simulink model "SAR_ADC_Dom_14_04_2017"  (R2016a)
settings: Solver=ode45  StartTime=0.0  StopTime=inf  FixedStep=1/255/2  RelTol=1e-3
libraries: simulink_extras x10
settings Model: Creator=ronip  LastModifiedBy=Lara
settings SolverCC: AutoInsertRateTranBlk=on
settings DataIOCC: SaveFormat=Array  SignalLoggingSaveFormat=ModelDataLogs  SaveOutput=off  SignalLogging=off  DSMLogging=off  SaveTime=off
settings OptimizationCC: ExpressionDepthLimit=2147483647  StateBitsets=on  DataBitsets=on  OptimizeModelRefInitCode=on  LifeSpan=1
settings DebuggingCC: UnderspecifiedInitializationDetection=Classic  MergeDetectMultiDrivingBlocksExec=none  SolverPrmCheckMsg=warning  FcnCallInpInsideContextMsg=UseLocalSettings  BusObjectLabelMismatch=error  StateNameClashWarn=warning
settings HardwareCC: ProdBitPerPointer=32  ProdLargestAtomicFloat=None  ProdIntDivRoundTo=Undefined  ProdEndianess=Unspecified  ProdWordSize=32  ProdHWDeviceType=32-bit Generic
settings ModelReferenceCC: PropagateSignalLabelsOutOfModel=off
settings RTWCC: SystemTargetFile=ert.tlc  TemplateMakefile=ert_default_tmf  Description=Real-Time Workshop Embedded Coder  GenerateReport=on  IncludeHyperlinkInReport=on  LaunchReport=on  CreateSILPILBlock=SIL  GenerateTraceInfo=on  GenerateTraceReport=on  GenerateTraceReportSl=on  GenerateTraceReportSf=on  GenerateTraceReportEml=on
settings CodeAppCC: IgnoreCustomStorageClasses=off  CustomSymbolStrType=$N$R$M  InternalIdentifier=Classic
settings ERTTargetCC: GenerateSampleERTMain=on  IncludeMdlTerminateFcn=off  ERTCustomFileTemplate=example_file_process.tlc  ConvertIfToSwitch=off  SuppressUnreachableDefaultCases=off
settings ConfigComp: CovModelRefEnable=Off

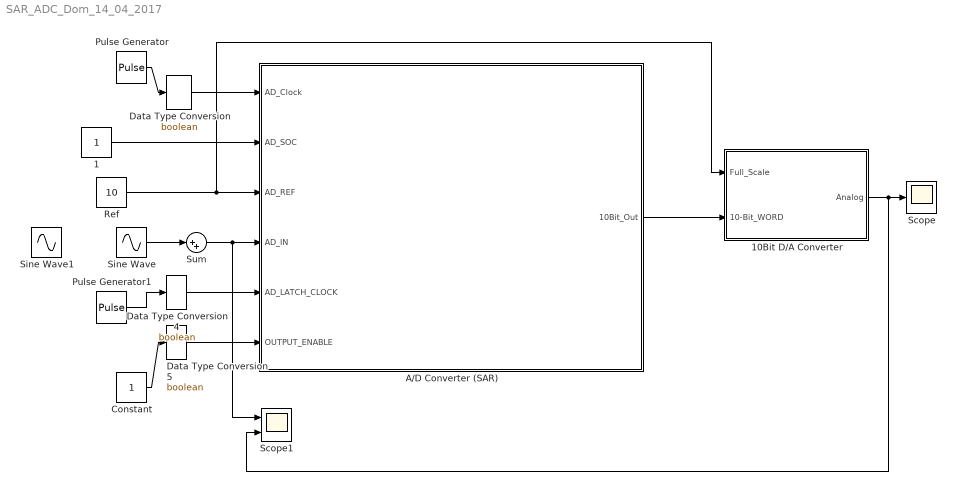
== system SAR_ADC_Dom_14_04_2017 ==
  1 : Constant
  10Bit D/A Converter : Subsystem  AncestorBlock=Digital_8bit_Library/8Bit D//A Converter
  A/D Converter (SAR) : Subsystem
      mask Display: disp('A/D Converter (SAR)')
  Constant : Constant
  Data Type Conversion : DataTypeConversion  OutDataTypeStr=boolean
  Data Type Conversion4 : DataTypeConversion  OutDataTypeStr=boolean
  Data Type Conversion5 : DataTypeConversion  OutDataTypeStr=boolean
  Pulse Generator : DiscretePulseGenerator  PulseType=Time based  Period=1/1023  PulseWidth=50
  Pulse Generator1 : DiscretePulseGenerator  PulseType=Time based  Period=0.001  PulseWidth=50
  Ref : Constant  Value=10
  Scope : Scope
  Scope1 : Scope  NumInputPorts=2
  Sine Wave : Sin  Amplitude=5  Bias=5  SampleTime=0
  Sine Wave1 : Sin  Amplitude=2  Bias=5  Frequency=4  SampleTime=0
  Sum : Sum  Inputs=|++
  wires:
  Constant/1 -> Data Type Conversion5/1
  Pulse Generator1/1 -> Data Type Conversion4/1
  Ref/1 -> A/D Converter (SAR)/3(AD_REF), 10Bit D/A Converter/1(Full_Scale)
  Pulse Generator/1 -> Data Type Conversion/1
  A/D Converter (SAR)/1(10Bit_Out) -> 10Bit D/A Converter/2(10-Bit_WORD)
  10Bit D/A Converter/1(Analog) -> Scope1/2, Scope/1
  Data Type Conversion/1 -> A/D Converter (SAR)/1(AD_Clock)
  1/1 -> A/D Converter (SAR)/2(AD_SOC)
  Data Type Conversion4/1 -> A/D Converter (SAR)/5(AD_LATCH_CLOCK)
  Data Type Conversion5/1 -> A/D Converter (SAR)/6(OUTPUT_ENABLE)
  Sum/1 -> Scope1/1, A/D Converter (SAR)/4(AD_IN)
  Sine Wave/1 -> Sum/1

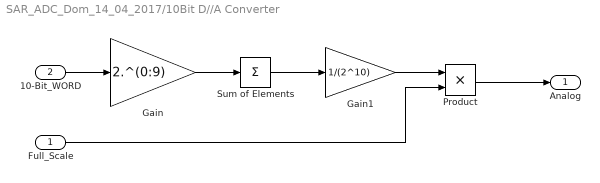
== system SAR_ADC_Dom_14_04_2017/10Bit D//A Converter ==
  Full_Scale : Inport
  10-Bit_WORD : Inport  Port=2
  Gain : Gain  Gain=2.^(0:9)
  Gain1 : Gain  Gain=1/(2^10)
  Product : Product  RndMeth=Zero
  Sum of Elements : Sum  Inputs=+
  Analog : Outport
  wires:
  10-Bit_WORD/1 -> Gain/1
  Full_Scale/1 -> Product/2
  Product/1 -> Analog/1
  Gain1/1 -> Product/1
  Sum of Elements/1 -> Gain1/1
  Gain/1 -> Sum of Elements/1

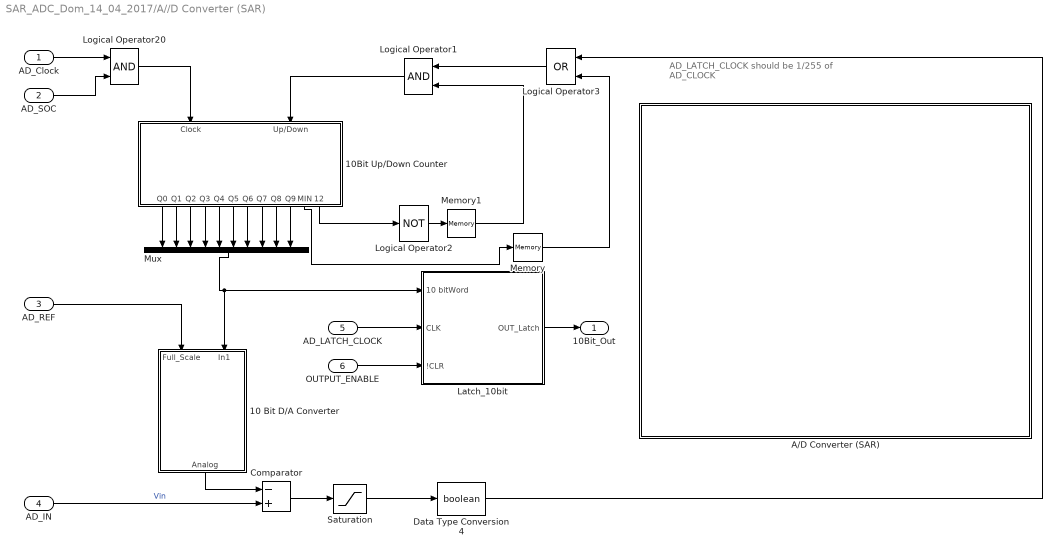
== system SAR_ADC_Dom_14_04_2017/A//D Converter (SAR) ==
  note: AD_LATCH_CLOCK should
      | be 1/255 of AD_CLOCK
  AD_Clock : Inport
  AD_SOC : Inport  Port=2
  AD_REF : Inport  Port=3
  AD_IN : Inport  Port=4
  AD_LATCH_CLOCK : Inport  Port=5
  OUTPUT_ENABLE : Inport  Port=6
  10 Bit D/A Converter : Subsystem  AncestorBlock=Digital_8bit_Library/8Bit D//A Converter
  10Bit Up/Down Counter : Subsystem  AncestorBlock="Digital_8bit_Library/8Bit Up//Down  Counter"
  A/D Converter (SAR) : Subsystem
      mask init:
      | maskImage= imread('A2D_SAR.jpg');
      mask Display: image(maskImage);
  Comparator : Sum  Inputs=-+  OutDataTypeStr=double
  Data Type Conversion4 : DataTypeConversion  OutDataTypeStr=boolean
  Latch_10bit : Subsystem  AncestorBlock=Digital_8bit_Library/Latch_8bit
  Logical Operator1 : Logic  IconShape=distinctive  AllPortsSameDT=off  OutDataTypeStr=boolean
  Logical Operator2 : Logic  Operator=NOT  IconShape=distinctive  AllPortsSameDT=off  OutDataTypeStr=boolean
  Logical Operator20 : Logic  IconShape=distinctive  AllPortsSameDT=off  OutDataTypeStr=boolean
  Logical Operator3 : Logic  Operator=OR  IconShape=distinctive  AllPortsSameDT=off  OutDataTypeStr=boolean
  Memory : Memory
  Memory1 : Memory
  Mux : Mux  Inputs=10
  Saturation : Saturate  UpperLimit=1  LowerLimit=0
  10Bit_Out : Outport
  wires:
  10Bit Up/Down Counter/7(Q6) -> Mux/7
  10Bit Up/Down Counter/1(Q0) -> Mux/1
  10Bit Up/Down Counter/2(Q1) -> Mux/2
  10Bit Up/Down Counter/3(Q2) -> Mux/3
  10Bit Up/Down Counter/4(Q3) -> Mux/4
  10Bit Up/Down Counter/5(Q4) -> Mux/5
  10Bit Up/Down Counter/6(Q5) -> Mux/6
  Mux/1 -> 10 Bit D/A Converter/2(In1), Latch_10bit/1(10 bitWord)
  Comparator/1 -> Saturation/1
  AD_Clock/1 -> Logical Operator20/1
  AD_REF/1 -> 10 Bit D/A Converter/1(Full_Scale)
  10 Bit D/A Converter/1(Analog) -> Comparator/1
  AD_IN/1 -> Comparator/2  "Vin"
  Saturation/1 -> Data Type Conversion4/1
  OUTPUT_ENABLE/1 -> Latch_10bit/3(!CLR)
  AD_SOC/1 -> Logical Operator20/2
  Logical Operator20/1 -> 10Bit Up/Down Counter/1(Clock)
  Latch_10bit/1(OUT_Latch) -> 10Bit_Out/1
  AD_LATCH_CLOCK/1 -> Latch_10bit/2(CLK)
  10Bit Up/Down Counter/12(MAX) -> Logical Operator2/1
  Logical Operator1/1 -> 10Bit Up/Down Counter/2(Up/Down)
  Data Type Conversion4/1 -> Logical Operator3/1
  10Bit Up/Down Counter/11(MIN) -> Memory/1
  Logical Operator2/1 -> Memory1/1
  Logical Operator3/1 -> Logical Operator1/1
  Memory1/1 -> Logical Operator1/2
  Memory/1 -> Logical Operator3/2
  10Bit Up/Down Counter/10(Q9) -> Mux/10
  10Bit Up/Down Counter/9(Q8) -> Mux/9
  10Bit Up/Down Counter/8(Q7) -> Mux/8

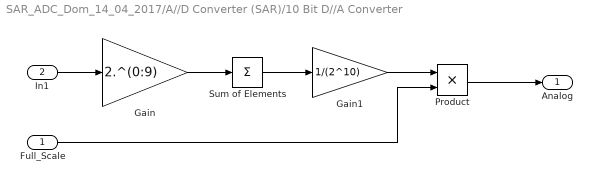
== system SAR_ADC_Dom_14_04_2017/A//D Converter (SAR)/10 Bit D//A Converter ==
  Full_Scale : Inport
  In1 : Inport  Port=2
  Gain : Gain  Gain=2.^(0:9)
  Gain1 : Gain  Gain=1/(2^10)
  Product : Product  RndMeth=Zero
  Sum of Elements : Sum  Inputs=+
  Analog : Outport
  wires:
  In1/1 -> Gain/1
  Full_Scale/1 -> Product/2
  Product/1 -> Analog/1
  Gain1/1 -> Product/1
  Sum of Elements/1 -> Gain1/1
  Gain/1 -> Sum of Elements/1

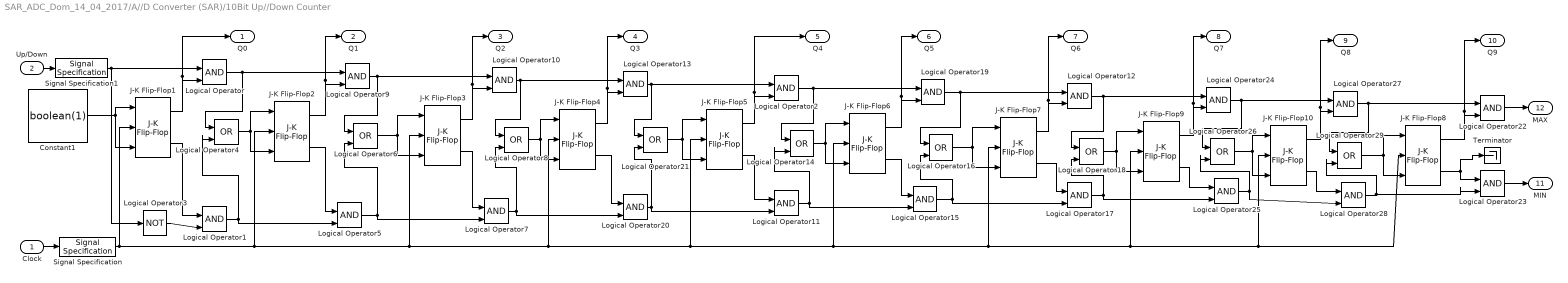
== system SAR_ADC_Dom_14_04_2017/A//D Converter (SAR)/10Bit Up//Down Counter ==
  Clock : Inport
  Up/Down : Inport  Port=2
  Constant1 : Constant  Value=boolean(1)
  J-K Flip-Flop{1..10} (10 alike) : simulink_extras/Flip Flops/J-K Flip-Flop  initial_condition=0
  Logical Operator{,1..2,5,7,9..13,15,17,19..20,22..25,27..28} (20 alike) : Logic  IconShape=distinctive  AllPortsSameDT=off  OutDataTypeStr=boolean
  Logical Operator{4,6,8,14,16,18,21,26,29} (9 alike) : Logic  Operator=OR  IconShape=distinctive  AllPortsSameDT=off  OutDataTypeStr=boolean
  Logical Operator3 : Logic  Operator=NOT  IconShape=distinctive  AllPortsSameDT=off  OutDataTypeStr=boolean
  Signal Specification : SignalSpecification  OutDataTypeStr=boolean
  Signal Specification1 : SignalSpecification  OutDataTypeStr=boolean
  Terminator : Terminator
  Q0 : Outport  InitialOutput=0
  Q1 : Outport  Port=2  InitialOutput=0
  Q2 : Outport  Port=3  InitialOutput=0
  Q3 : Outport  Port=4  InitialOutput=0
  Q4 : Outport  Port=5  InitialOutput=0
  Q5 : Outport  Port=6  InitialOutput=0
  Q6 : Outport  Port=7  InitialOutput=0
  Q7 : Outport  Port=8  InitialOutput=0
  Q8 : Outport  Port=9  InitialOutput=0
  Q9 : Outport  Port=10  InitialOutput=0
  MIN : Outport  Port=11  InitialOutput=0
  MAX : Outport  Port=12  InitialOutput=0
  wires:
  Signal Specification1/1 -> Logical Operator/1, Logical Operator3/1
  Logical Operator21/1 -> J-K Flip-Flop5/3, J-K Flip-Flop5/1
  Logical Operator20/1 -> Logical Operator11/2, Logical Operator21/2
  Logical Operator13/1 -> Logical Operator2/1, Logical Operator21/1
  Logical Operator12/1 -> Logical Operator18/1, Logical Operator24/1
  Logical Operator19/1 -> Logical Operator12/1, Logical Operator16/1
  Logical Operator17/1 -> Logical Operator25/2, Logical Operator18/2
  Logical Operator15/1 -> Logical Operator17/2, Logical Operator16/2
  Logical Operator16/1 -> J-K Flip-Flop7/3, J-K Flip-Flop7/1
  Logical Operator11/1 -> Logical Operator15/2, Logical Operator14/2
  Logical Operator14/1 -> J-K Flip-Flop6/3, J-K Flip-Flop6/1
  J-K Flip-Flop6/1 -> Q5/1, Logical Operator19/2
  J-K Flip-Flop7/1 -> Q6/1, Logical Operator12/2
  J-K Flip-Flop7/2 -> Logical Operator17/1
  Logical Operator2/1 -> Logical Operator19/1, Logical Operator14/1
  J-K Flip-Flop5/1 -> Q4/1, Logical Operator2/2
  J-K Flip-Flop5/2 -> Logical Operator11/1
  J-K Flip-Flop6/2 -> Logical Operator15/1
  Logical Operator10/1 -> Logical Operator13/1, Logical Operator8/1
  Logical Operator9/1 -> Logical Operator10/1, Logical Operator6/1
  Logical Operator8/1 -> J-K Flip-Flop4/3, J-K Flip-Flop4/1
  Logical Operator7/1 -> Logical Operator20/2, Logical Operator8/2
  Logical Operator5/1 -> Logical Operator7/2, Logical Operator6/2
  Logical Operator6/1 -> J-K Flip-Flop3/3, J-K Flip-Flop3/1
  Logical Operator4/1 -> J-K Flip-Flop2/1, J-K Flip-Flop2/3
  J-K Flip-Flop2/1 -> Q1/1, Logical Operator9/2
  J-K Flip-Flop4/1 -> Q3/1, Logical Operator13/2
  J-K Flip-Flop3/1 -> Q2/1, Logical Operator10/2
  J-K Flip-Flop3/2 -> Logical Operator7/1
  J-K Flip-Flop4/2 -> Logical Operator20/1
  J-K Flip-Flop2/2 -> Logical Operator5/1
  J-K Flip-Flop8/1 -> Q9/1, Logical Operator22/2
  J-K Flip-Flop8/2 -> Terminator/1, Logical Operator23/1
  Logical Operator1/1 -> Logical Operator5/2, Logical Operator4/2
  Logical Operator3/1 -> Logical Operator1/2
  Up/Down/1 -> Signal Specification1/1
  Constant1/1 -> J-K Flip-Flop1/1, J-K Flip-Flop1/3
  Clock/1 -> Signal Specification/1
  Logical Operator/1 -> Logical Operator9/1, Logical Operator4/1
  J-K Flip-Flop1/1 -> Logical Operator/2, Q0/1
  J-K Flip-Flop1/2 -> Logical Operator1/1
  Logical Operator22/1 -> MAX/1
  Logical Operator23/1 -> MIN/1
  Logical Operator18/1 -> J-K Flip-Flop9/3, J-K Flip-Flop9/1
  J-K Flip-Flop9/1 -> Logical Operator24/2, Q7/1
  J-K Flip-Flop9/2 -> Logical Operator25/1
  Logical Operator24/1 -> Logical Operator26/1, Logical Operator27/1
  Logical Operator25/1 -> Logical Operator28/2, Logical Operator26/2
  J-K Flip-Flop10/1 -> Logical Operator27/2, Q8/1
  Logical Operator27/1 -> Logical Operator22/1, Logical Operator29/1
  Logical Operator28/1 -> Logical Operator23/2, Logical Operator29/2
  J-K Flip-Flop10/2 -> Logical Operator28/1
  Logical Operator26/1 -> J-K Flip-Flop10/3, J-K Flip-Flop10/1
  Signal Specification/1 -> J-K Flip-Flop3/2, J-K Flip-Flop4/2, J-K Flip-Flop5/2, J-K Flip-Flop6/2, J-K Flip-Flop9/2, J-K Flip-Flop8/2, J-K Flip-Flop10/2, J-K Flip-Flop7/2, J-K Flip-Flop2/2, J-K Flip-Flop1/2
  Logical Operator29/1 -> J-K Flip-Flop8/3, J-K Flip-Flop8/1

== system SAR_ADC_Dom_14_04_2017/A//D Converter (SAR)/A//D Converter (SAR) ==

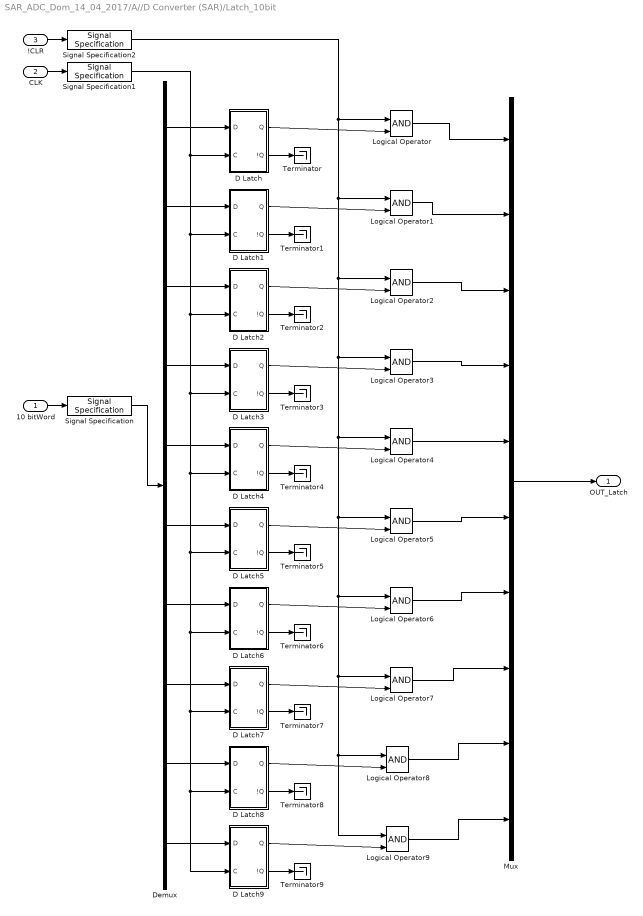
== system SAR_ADC_Dom_14_04_2017/A//D Converter (SAR)/Latch_10bit ==
  10 bitWord : Inport
  CLK : Inport  Port=2
  !CLR : Inport  Port=3
  D Latch : Subsystem  mask(DLatch){}
      mask help: D Latch Flip-Flop Block
      mask Help: web([docroot '/toolbox/simulink/ref_extras/dlatch.html'])
  D Latch1 : Subsystem  mask(DLatch){}
      mask help: D Latch Flip-Flop Block
      mask Help: web([docroot '/toolbox/simulink/ref_extras/dlatch.html'])
  D Latch2 : Subsystem  mask(DLatch){}
      mask help: D Latch Flip-Flop Block
      mask Help: web([docroot '/toolbox/simulink/ref_extras/dlatch.html'])
  D Latch3 : Subsystem  mask(DLatch){}
      mask help: D Latch Flip-Flop Block
      mask Help: web([docroot '/toolbox/simulink/ref_extras/dlatch.html'])
  D Latch4 : Subsystem  mask(DLatch){}
      mask help: D Latch Flip-Flop Block
      mask Help: web([docroot '/toolbox/simulink/ref_extras/dlatch.html'])
  D Latch5 : Subsystem  mask(DLatch){}
      mask help: D Latch Flip-Flop Block
      mask Help: web([docroot '/toolbox/simulink/ref_extras/dlatch.html'])
  D Latch6 : Subsystem  mask(DLatch){}
      mask help: D Latch Flip-Flop Block
      mask Help: web([docroot '/toolbox/simulink/ref_extras/dlatch.html'])
  D Latch7 : Subsystem  mask(DLatch){}
      mask help: D Latch Flip-Flop Block
      mask Help: web([docroot '/toolbox/simulink/ref_extras/dlatch.html'])
  D Latch8 : Subsystem  mask(DLatch){}
      mask help: D Latch Flip-Flop Block
      mask Help: web([docroot '/toolbox/simulink/ref_extras/dlatch.html'])
  D Latch9 : Subsystem  mask(DLatch){}
      mask help: D Latch Flip-Flop Block
      mask Help: web([docroot '/toolbox/simulink/ref_extras/dlatch.html'])
  Demux : Demux  Outputs=10
  Logical Operator{,1..9} (10 alike) : Logic  IconShape=distinctive  AllPortsSameDT=off  OutDataTypeStr=boolean
  Mux : Mux  Inputs=10
  Signal Specification : SignalSpecification  OutDataTypeStr=boolean
  Signal Specification1 : SignalSpecification  OutDataTypeStr=boolean
  Signal Specification2 : SignalSpecification  OutDataTypeStr=boolean
  Terminator{,1..9} (10 alike) : Terminator
  OUT_Latch : Outport
  wires:
  10 bitWord/1 -> Signal Specification/1
  CLK/1 -> Signal Specification1/1
  D Latch/2(!Q) -> Terminator/1
  D Latch1/2(!Q) -> Terminator1/1
  D Latch2/2(!Q) -> Terminator2/1
  D Latch3/2(!Q) -> Terminator3/1
  D Latch4/2(!Q) -> Terminator4/1
  D Latch5/2(!Q) -> Terminator5/1
  D Latch6/2(!Q) -> Terminator6/1
  D Latch7/2(!Q) -> Terminator7/1
  Demux/1 -> D Latch/1(D)
  Demux/2 -> D Latch1/1(D)
  Demux/3 -> D Latch2/1(D)
  Demux/4 -> D Latch3/1(D)
  Demux/5 -> D Latch4/1(D)
  Demux/6 -> D Latch5/1(D)
  Demux/7 -> D Latch6/1(D)
  Demux/8 -> D Latch7/1(D)
  D Latch1/1(Q) -> Logical Operator1/2
  D Latch2/1(Q) -> Logical Operator2/2
  D Latch3/1(Q) -> Logical Operator3/2
  D Latch6/1(Q) -> Logical Operator6/2
  D Latch7/1(Q) -> Logical Operator7/2
  Mux/1 -> OUT_Latch/1
  !CLR/1 -> Signal Specification2/1
  D Latch5/1(Q) -> Logical Operator5/2
  D Latch4/1(Q) -> Logical Operator4/2
  Logical Operator/1 -> Mux/1
  Logical Operator1/1 -> Mux/2
  Logical Operator2/1 -> Mux/3
  Logical Operator3/1 -> Mux/4
  Logical Operator4/1 -> Mux/5
  Logical Operator5/1 -> Mux/6
  Logical Operator6/1 -> Mux/7
  Logical Operator7/1 -> Mux/8
  D Latch/1(Q) -> Logical Operator/2
  Signal Specification/1 -> Demux/1
  Signal Specification1/1 -> D Latch6/2(C), D Latch9/2(C), D Latch8/2(C), D Latch7/2(C), D Latch5/2(C), D Latch4/2(C), D Latch3/2(C), D Latch2/2(C), D Latch1/2(C), D Latch/2(C)
  Signal Specification2/1 -> Logical Operator1/1, Logical Operator2/1, Logical Operator3/1, Logical Operator4/1, Logical Operator9/1, Logical Operator8/1, Logical Operator7/1, Logical Operator6/1, Logical Operator5/1, Logical Operator/1
  Demux/9 -> D Latch8/1(D)
  Demux/10 -> D Latch9/1(D)
  D Latch9/2(!Q) -> Terminator9/1
  D Latch8/2(!Q) -> Terminator8/1
  Logical Operator8/1 -> Mux/9
  Logical Operator9/1 -> Mux/10
  D Latch8/1(Q) -> Logical Operator8/2
  D Latch9/1(Q) -> Logical Operator9/2

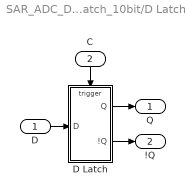
== system SAR_ADC_Dom_14_04_2017/A//D Converter (SAR)/Latch_10bit/D Latch ==
  D : Inport
  C : Inport  Port=2
  D Latch : Subsystem  TreatAsAtomicUnit=on
  Q : Outport  InitialOutput=0
  !Q : Outport  Port=2  InitialOutput=1
  wires:
  C/1 -> D Latch/Trigger
  D Latch/1(Q) -> Q/1
  D/1 -> D Latch/1(D)
  D Latch/2(!Q) -> !Q/1

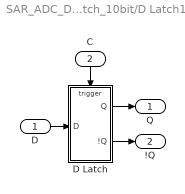
== system SAR_ADC_Dom_14_04_2017/A//D Converter (SAR)/Latch_10bit/D Latch1 ==
  D : Inport
  C : Inport  Port=2
  D Latch : Subsystem  TreatAsAtomicUnit=on
  Q : Outport  InitialOutput=0
  !Q : Outport  Port=2  InitialOutput=1
  wires:
  D Latch/2(!Q) -> !Q/1
  D/1 -> D Latch/1(D)
  D Latch/1(Q) -> Q/1
  C/1 -> D Latch/Trigger

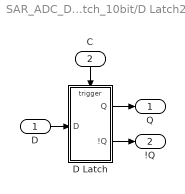
== system SAR_ADC_Dom_14_04_2017/A//D Converter (SAR)/Latch_10bit/D Latch2 ==
  D : Inport
  C : Inport  Port=2
  D Latch : Subsystem  TreatAsAtomicUnit=on
  Q : Outport  InitialOutput=0
  !Q : Outport  Port=2  InitialOutput=1
  wires:
  C/1 -> D Latch/Trigger
  D Latch/1(Q) -> Q/1
  D/1 -> D Latch/1(D)
  D Latch/2(!Q) -> !Q/1

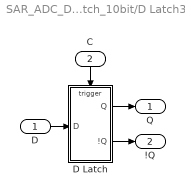
== system SAR_ADC_Dom_14_04_2017/A//D Converter (SAR)/Latch_10bit/D Latch3 ==
  D : Inport
  C : Inport  Port=2
  D Latch : Subsystem  TreatAsAtomicUnit=on
  Q : Outport  InitialOutput=0
  !Q : Outport  Port=2  InitialOutput=1
  wires:
  D Latch/2(!Q) -> !Q/1
  D/1 -> D Latch/1(D)
  D Latch/1(Q) -> Q/1
  C/1 -> D Latch/Trigger

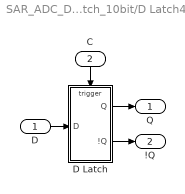
== system SAR_ADC_Dom_14_04_2017/A//D Converter (SAR)/Latch_10bit/D Latch4 ==
  D : Inport
  C : Inport  Port=2
  D Latch : Subsystem  TreatAsAtomicUnit=on
  Q : Outport  InitialOutput=0
  !Q : Outport  Port=2  InitialOutput=1
  wires:
  C/1 -> D Latch/Trigger
  D Latch/1(Q) -> Q/1
  D/1 -> D Latch/1(D)
  D Latch/2(!Q) -> !Q/1

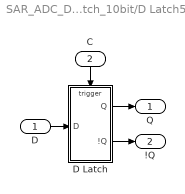
== system SAR_ADC_Dom_14_04_2017/A//D Converter (SAR)/Latch_10bit/D Latch5 ==
  D : Inport
  C : Inport  Port=2
  D Latch : Subsystem  TreatAsAtomicUnit=on
  Q : Outport  InitialOutput=0
  !Q : Outport  Port=2  InitialOutput=1
  wires:
  D Latch/2(!Q) -> !Q/1
  D/1 -> D Latch/1(D)
  D Latch/1(Q) -> Q/1
  C/1 -> D Latch/Trigger

== system SAR_ADC_Dom_14_04_2017/A//D Converter (SAR)/Latch_10bit/D Latch6 ==
  D : Inport
  C : Inport  Port=2
  D Latch : Subsystem  TreatAsAtomicUnit=on
  Q : Outport  InitialOutput=0
  !Q : Outport  Port=2  InitialOutput=1
  wires:
  C/1 -> D Latch/Trigger
  D Latch/1(Q) -> Q/1
  D/1 -> D Latch/1(D)
  D Latch/2(!Q) -> !Q/1

== system SAR_ADC_Dom_14_04_2017/A//D Converter (SAR)/Latch_10bit/D Latch7 ==
  D : Inport
  C : Inport  Port=2
  D Latch : Subsystem  TreatAsAtomicUnit=on
  Q : Outport  InitialOutput=0
  !Q : Outport  Port=2  InitialOutput=1
  wires:
  D Latch/2(!Q) -> !Q/1
  D/1 -> D Latch/1(D)
  D Latch/1(Q) -> Q/1
  C/1 -> D Latch/Trigger

== system SAR_ADC_Dom_14_04_2017/A//D Converter (SAR)/Latch_10bit/D Latch8 ==
  D : Inport
  C : Inport  Port=2
  D Latch : Subsystem  TreatAsAtomicUnit=on
  Q : Outport  InitialOutput=0
  !Q : Outport  Port=2  InitialOutput=1
  wires:
  D Latch/2(!Q) -> !Q/1
  D/1 -> D Latch/1(D)
  D Latch/1(Q) -> Q/1
  C/1 -> D Latch/Trigger

== system SAR_ADC_Dom_14_04_2017/A//D Converter (SAR)/Latch_10bit/D Latch9 ==
  D : Inport
  C : Inport  Port=2
  D Latch : Subsystem  TreatAsAtomicUnit=on
  Q : Outport  InitialOutput=0
  !Q : Outport  Port=2  InitialOutput=1
  wires:
  D Latch/2(!Q) -> !Q/1
  D/1 -> D Latch/1(D)
  D Latch/1(Q) -> Q/1
  C/1 -> D Latch/Trigger

== system SAR_ADC_Dom_14_04_2017/A//D Converter (SAR)/Latch_10bit/D Latch/D Latch ==
  D : Inport
  Trigger : TriggerPort  VariantControl=Variant
  Logic : Logic  Operator=NOT  Inputs=1
  Q : Outport  InitialOutput=0
  !Q : Outport  Port=2  InitialOutput=1
  wires:
  Logic/1 -> !Q/1
  D/1 -> Q/1, Logic/1

== system SAR_ADC_Dom_14_04_2017/A//D Converter (SAR)/Latch_10bit/D Latch1/D Latch ==
  D : Inport
  Trigger : TriggerPort  VariantControl=Variant
  Logic : Logic  Operator=NOT  Inputs=1
  Q : Outport  InitialOutput=0
  !Q : Outport  Port=2  InitialOutput=1
  wires:
  D/1 -> Logic/1, Q/1
  Logic/1 -> !Q/1

== system SAR_ADC_Dom_14_04_2017/A//D Converter (SAR)/Latch_10bit/D Latch2/D Latch ==
  D : Inport
  Trigger : TriggerPort  VariantControl=Variant
  Logic : Logic  Operator=NOT  Inputs=1
  Q : Outport  InitialOutput=0
  !Q : Outport  Port=2  InitialOutput=1
  wires:
  Logic/1 -> !Q/1
  D/1 -> Q/1, Logic/1

== system SAR_ADC_Dom_14_04_2017/A//D Converter (SAR)/Latch_10bit/D Latch3/D Latch ==
  D : Inport
  Trigger : TriggerPort  VariantControl=Variant
  Logic : Logic  Operator=NOT  Inputs=1
  Q : Outport  InitialOutput=0
  !Q : Outport  Port=2  InitialOutput=1
  wires:
  D/1 -> Logic/1, Q/1
  Logic/1 -> !Q/1

== system SAR_ADC_Dom_14_04_2017/A//D Converter (SAR)/Latch_10bit/D Latch4/D Latch ==
  D : Inport
  Trigger : TriggerPort  VariantControl=Variant
  Logic : Logic  Operator=NOT  Inputs=1
  Q : Outport  InitialOutput=0
  !Q : Outport  Port=2  InitialOutput=1
  wires:
  Logic/1 -> !Q/1
  D/1 -> Q/1, Logic/1

== system SAR_ADC_Dom_14_04_2017/A//D Converter (SAR)/Latch_10bit/D Latch5/D Latch ==
  D : Inport
  Trigger : TriggerPort  VariantControl=Variant
  Logic : Logic  Operator=NOT  Inputs=1
  Q : Outport  InitialOutput=0
  !Q : Outport  Port=2  InitialOutput=1
  wires:
  D/1 -> Logic/1, Q/1
  Logic/1 -> !Q/1

== system SAR_ADC_Dom_14_04_2017/A//D Converter (SAR)/Latch_10bit/D Latch6/D Latch ==
  D : Inport
  Trigger : TriggerPort  VariantControl=Variant
  Logic : Logic  Operator=NOT  Inputs=1
  Q : Outport  InitialOutput=0
  !Q : Outport  Port=2  InitialOutput=1
  wires:
  Logic/1 -> !Q/1
  D/1 -> Q/1, Logic/1

== system SAR_ADC_Dom_14_04_2017/A//D Converter (SAR)/Latch_10bit/D Latch7/D Latch ==
  D : Inport
  Trigger : TriggerPort  VariantControl=Variant
  Logic : Logic  Operator=NOT  Inputs=1
  Q : Outport  InitialOutput=0
  !Q : Outport  Port=2  InitialOutput=1
  wires:
  D/1 -> Logic/1, Q/1
  Logic/1 -> !Q/1

== system SAR_ADC_Dom_14_04_2017/A//D Converter (SAR)/Latch_10bit/D Latch8/D Latch ==
  D : Inport
  Trigger : TriggerPort  VariantControl=Variant
  Logic : Logic  Operator=NOT  Inputs=1
  Q : Outport  InitialOutput=0
  !Q : Outport  Port=2  InitialOutput=1
  wires:
  D/1 -> Logic/1, Q/1
  Logic/1 -> !Q/1

== system SAR_ADC_Dom_14_04_2017/A//D Converter (SAR)/Latch_10bit/D Latch9/D Latch ==
  D : Inport
  Trigger : TriggerPort  VariantControl=Variant
  Logic : Logic  Operator=NOT  Inputs=1
  Q : Outport  InitialOutput=0
  !Q : Outport  Port=2  InitialOutput=1
  wires:
  D/1 -> Logic/1, Q/1
  Logic/1 -> !Q/1
